simulink library "DCDC"  (R2025a)
settings: Solver=VariableStepAuto  StartTime=0.0  StopTime=10.0  RelTol=1e-3
undefined symbols (not defined in the file or in its folder): raptor_xcp_function, StateCAN
libraries: Utilities x18, Raptor_lib x2, simulink x1
settings Model: Creator=serga  LastModifiedBy=hyuga

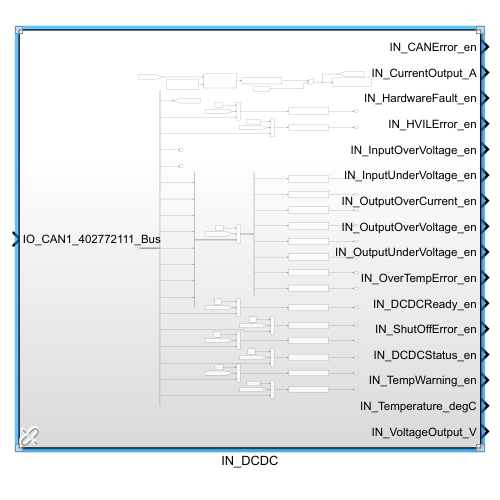
[thumbnail: Simulink's stored preview of the top-level diagram]
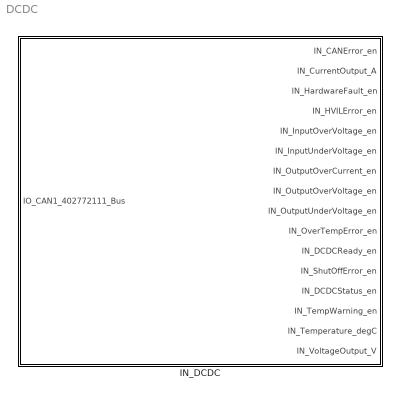
== system DCDC ==
  IN_DCDC : Subsystem  AncestorBlock=DCDC/IN_DCDC

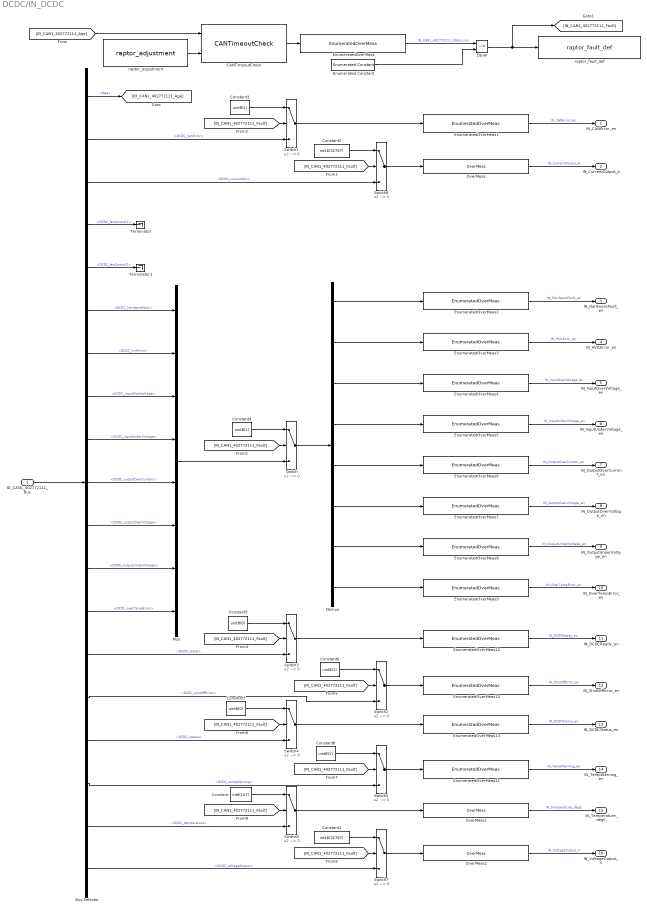
== system DCDC/IN_DCDC ==
  IO_CAN1_402772111_Bus : Inport
  Bus Selector : BusSelector  OutputSignals=Age,DCDC_canError,DCDC_currentOut,DCDC_fanControl1,DCDC_fanControl2,DCDC_hardwarefault,DCDC_hvilError,DCDC_inputOverVoltage,DCDC_inputUnderVoltage,DCDC_outputOverCurrent,DCDC_outputOverVoltage,DCDC_outputUnderVoltage,DCDC_overTempError,DCDC_ready,DCDC_shutOffError,DCDC_status,DCDC_tempWarning,DCDC_temperature,DCDC_voltageOutput
  CANTimeoutCheck : Utilities/CANTimeoutCheck
  Constant : Constant  Value=int8(127)
  Constant1 : Constant  Value=int16(32767)
  Constant2 : Constant  Value=int16(32767)
  Constant{3..4,6,8} (4 alike) : Constant  Value=uint8(1)
  Constant5 : Constant  Value=uint8(0)
  Constant7 : Constant  Value=uint8(0)
  Demux : Demux  Outputs=8
  Enumerated Constant : simulink/Sources/Enumerated Constant  OutDataTypeStr=Enum: StateCAN  Value=StateCAN.Normal  SampleTime=inf
  EnumeratedOverMeas : Utilities/EnumeratedOverMeas  sigName='IN_CAN1_402772111_Status_en'  enumName='StateCAN'
  EnumeratedOverMeas1 : Utilities/EnumeratedOverMeas  sigName='IN_CANError_en'  enumName='DCDCFaultState'
  EnumeratedOverMeas10 : Utilities/EnumeratedOverMeas  sigName='IN_ShutOffError_en'  enumName='DCDCFaultState'
  EnumeratedOverMeas11 : Utilities/EnumeratedOverMeas  sigName='IN_TempWarning_en'  enumName='DCDCFaultState'
  EnumeratedOverMeas12 : Utilities/EnumeratedOverMeas  sigName='IN_DCDCReady_en'  enumName='DCDCStatus'
  EnumeratedOverMeas13 : Utilities/EnumeratedOverMeas  sigName='IN_DCDCStatus_en'  enumName='DCDCStatus'
  EnumeratedOverMeas2 : Utilities/EnumeratedOverMeas  sigName='IN_HardwareFault_en'  enumName='DCDCFaultState'
  EnumeratedOverMeas3 : Utilities/EnumeratedOverMeas  sigName='IN_HVILError_en'  enumName='DCDCFaultState'
  EnumeratedOverMeas4 : Utilities/EnumeratedOverMeas  sigName='IN_InputOverVoltage_en'  enumName='DCDCFaultState'
  EnumeratedOverMeas5 : Utilities/EnumeratedOverMeas  sigName='IN_InputUnderVoltage_en'  enumName='DCDCFaultState'
  EnumeratedOverMeas6 : Utilities/EnumeratedOverMeas  sigName='IN_OutputOverCurrent_en'  enumName='DCDCFaultState'
  EnumeratedOverMeas7 : Utilities/EnumeratedOverMeas  sigName='IN_OutputOverVoltage_en'  enumName='DCDCFaultState'
  EnumeratedOverMeas8 : Utilities/EnumeratedOverMeas  sigName='IN_OutputUnderVoltage_en'  enumName='DCDCFaultState'
  EnumeratedOverMeas9 : Utilities/EnumeratedOverMeas  sigName='IN_OverTempError_en'  enumName='DCDCFaultState'
  Equal : RelationalOperator  Operator=~=  OutDataTypeStr=boolean  RndMeth=Simplest  InputSameDT=off
  Mux : Mux  Inputs=8
  OverMeas : Utilities/OverMeas  sigName='IN_CurrentOutput_A'  minimum=-inf  maximum=inf
  OverMeas1 : Utilities/OverMeas  sigName='IN_Temperature_degC'  minimum=-inf  maximum=inf
  OverMeas2 : Utilities/OverMeas  sigName='IN_VoltageOutput_V'  minimum=-inf  maximum=inf
  Switch{,1..8} (9 alike) : Switch  Criteria=u2 ~= 0  SaturateOnIntegerOverflow=off  InputSameDT=off
  Terminator : Terminator
  Terminator1 : Terminator
  raptor_adjustment : Raptor_lib/Data Storage/raptor_adjustment  paramName='IN_DCDCTOThresh_na'  nameSource=Parameter  initValue=20  dataType=uint32  storage=Calibration  calDispType=Number  calEnum={'False', 'True'}  calGain=1.0  calOffset=0.0  calMax=inf  calMin=-inf  calFormat='-1'  calUnit=''  calHelp=''  calAccess=1  calFunction=raptor_xcp_function(gcb)  calDispHeaders=off  calColHeaders={'Col1' 'Col2' 'Col3'}  calRowHeaders={'Row1' 'Row2' 'Row3'}
      settings: SourceProductName=Raptor
  raptor_fault_def : Raptor_lib/Faults/raptor_fault_def  faultName='IN_CAN1_402772111_Fault'  persist=on  sticky=off  emisRelated=off  permanent=off  singleTrip=off  clearMethod=Standard  xLimit=25  yLimit=50  calEnable=on  addDisable=off  calAccess=1  calFunction='System | FaultManager'
      settings: SourceProductName=Raptor
  IN_CANError_en : Outport
  IN_CurrentOutput_A : Outport  Port=2
  IN_HardwareFault_en : Outport  Port=3
  IN_HVILError_en : Outport  Port=4
  IN_InputOverVoltage_en : Outport  Port=5
  IN_InputUnderVoltage_en : Outport  Port=6
  IN_OutputOverCurrent_en : Outport  Port=7
  IN_OutputOverVoltage_en : Outport  Port=8
  IN_OutputUnderVoltage_en : Outport  Port=9
  IN_OverTempError_en : Outport  Port=10
  IN_DCDCReady_en : Outport  Port=11
  IN_ShutOffError_en : Outport  Port=12
  IN_DCDCStatus_en : Outport  Port=13
  IN_TempWarning_en : Outport  Port=14
  IN_Temperature_degC : Outport  Port=15
  IN_VoltageOutput_V : Outport  Port=16
  wires:
  Bus Selector/3 -> Switch8/3  "<DCDC_currentOut>"
  IO_CAN1_402772111_Bus/1 -> Bus Selector/1
  Bus Selector/1 -> [IO_CAN1_402772111_Age]  "<Age>"
  Bus Selector/2 -> Switch1/3  "<DCDC_canError>"
  Bus Selector/4 -> Terminator/1  "<DCDC_fanControl1>"
  Bus Selector/5 -> Terminator1/1  "<DCDC_fanControl2>"
  Bus Selector/7 -> Mux/2  "<DCDC_hvilError>"
  Bus Selector/8 -> Mux/3  "<DCDC_inputOverVoltage>"
  Bus Selector/9 -> Mux/4  "<DCDC_inputUnderVoltage>"
  Bus Selector/10 -> Mux/5  "<DCDC_outputOverCurrent>"
  Bus Selector/11 -> Mux/6  "<DCDC_outputOverVoltage>"
  Bus Selector/12 -> Mux/7  "<DCDC_outputUnderVoltage>"
  Bus Selector/13 -> Mux/8  "<DCDC_overTempError>"
  Bus Selector/14 -> Switch3/3  "<DCDC_ready>"
  Bus Selector/15 -> Switch2/3  "<DCDC_shutOffError>"
  Bus Selector/16 -> Switch4/3  "<DCDC_status>"
  Bus Selector/17 -> Switch5/3  "<DCDC_tempWarning>"
  Bus Selector/18 -> Switch6/3  "<DCDC_temperature>"
  Bus Selector/19 -> Switch7/3  "<DCDC_voltageOutput>"
  [IO_CAN1_402772111_Age] -> CANTimeoutCheck/1
  raptor_adjustment/1 -> CANTimeoutCheck/2
  CANTimeoutCheck/1 -> EnumeratedOverMeas/1
  EnumeratedOverMeas/1 -> Equal/1  "IN_CAN1_402772111_Status_en"
  Enumerated Constant/1 -> Equal/2
  Equal/1 -> [IN_CAN1_402772111_Fault], raptor_fault_def/1
  Mux/1 -> Switch/3
  [IN_CAN1_402772111_Fault] -> Switch/2
  [IN_CAN1_402772111_Fault] -> Switch1/2
  Constant3/1 -> Switch1/1
  [IN_CAN1_402772111_Fault] -> Switch8/2
  [IN_CAN1_402772111_Fault] -> Switch3/2
  [IN_CAN1_402772111_Fault] -> Switch2/2
  [IN_CAN1_402772111_Fault] -> Switch4/2
  [IN_CAN1_402772111_Fault] -> Switch5/2
  [IN_CAN1_402772111_Fault] -> Switch6/2
  [IN_CAN1_402772111_Fault] -> Switch7/2
  Constant6/1 -> Switch2/1
  Constant8/1 -> Switch5/1
  Constant5/1 -> Switch3/1
  Constant7/1 -> Switch4/1
  Constant/1 -> Switch6/1
  Constant1/1 -> Switch7/1
  Constant2/1 -> Switch8/1
  Switch1/1 -> EnumeratedOverMeas1/1
  Switch/1 -> Demux/1
  Demux/1 -> EnumeratedOverMeas2/1
  Demux/2 -> EnumeratedOverMeas3/1
  Demux/3 -> EnumeratedOverMeas4/1
  Demux/4 -> EnumeratedOverMeas5/1
  Demux/5 -> EnumeratedOverMeas6/1
  Demux/6 -> EnumeratedOverMeas7/1
  Demux/7 -> EnumeratedOverMeas8/1
  Demux/8 -> EnumeratedOverMeas9/1
  Switch2/1 -> EnumeratedOverMeas10/1
  Switch5/1 -> EnumeratedOverMeas11/1
  Switch3/1 -> EnumeratedOverMeas12/1
  Switch4/1 -> EnumeratedOverMeas13/1
  Switch8/1 -> OverMeas/1
  Switch6/1 -> OverMeas1/1
  Switch7/1 -> OverMeas2/1
  EnumeratedOverMeas1/1 -> IN_CANError_en/1  "IN_CANError_en"
  OverMeas/1 -> IN_CurrentOutput_A/1  "IN_CurrentOutput_A"
  EnumeratedOverMeas2/1 -> IN_HardwareFault_en/1  "IN_HardwareFault_en"
  EnumeratedOverMeas3/1 -> IN_HVILError_en/1  "IN_HVILError_en"
  EnumeratedOverMeas4/1 -> IN_InputOverVoltage_en/1  "IN_InputOverVoltage_en"
  EnumeratedOverMeas5/1 -> IN_InputUnderVoltage_en/1  "IN_InputUnderVoltage_en"
  EnumeratedOverMeas6/1 -> IN_OutputOverCurrent_en/1  "IN_OutputOverCurrent_en"
  EnumeratedOverMeas7/1 -> IN_OutputOverVoltage_en/1  "IN_OutputOverVoltage_en"
  EnumeratedOverMeas8/1 -> IN_OutputUnderVoltage_en/1  "IN_OutputUnderVoltage_en"
  EnumeratedOverMeas9/1 -> IN_OverTempError_en/1  "IN_OverTempError_en"
  EnumeratedOverMeas12/1 -> IN_DCDCReady_en/1  "IN_DCDCReady_en"
  EnumeratedOverMeas10/1 -> IN_ShutOffError_en/1  "IN_ShutOffError_en"
  EnumeratedOverMeas13/1 -> IN_DCDCStatus_en/1  "IN_DCDCStatus_en"
  EnumeratedOverMeas11/1 -> IN_TempWarning_en/1  "IN_TempWarning_en"
  OverMeas1/1 -> IN_Temperature_degC/1  "IN_Temperature_degC"
  OverMeas2/1 -> IN_VoltageOutput_V/1  "IN_VoltageOutput_V"
  Constant4/1 -> Switch/1
  Bus Selector/6 -> Mux/1  "<DCDC_hardwarefault>"
